simulink model "myMotor"  (R2020a)
settings: Solver=FixedStepAuto  StartTime=0.0  StopTime=10  FixedStep=0.005  RelTol=1e-3
values from neighbouring files (symbols this model uses):
  B = 6.60509857261e-05    [myNewMotor.mat]
  J = 3.18348551573e-05    [myNewMotor.mat]
  K = 0.0751678132976    [myNewMotor.mat]
  L = 0.0712541882931    [myNewMotor.mat]
  R = 6.4    [myNewMotor.mat]
settings Model: OrderedModelArguments=off  Creator=sabir  LastModifiedBy=sabir

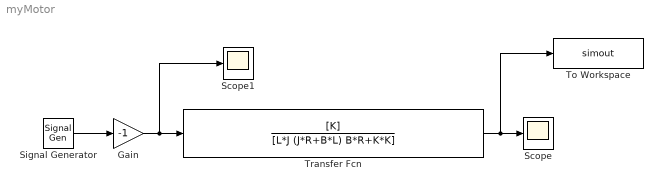
== system myMotor ==
  Gain : Gain  Gain=-1
  Scope : Scope
  Scope1 : Scope
  Signal Generator : SignalGenerator  WaveForm=square  Amplitude=24  Frequency=0.5
  To Workspace : ToWorkspace  VariableName=simout  SampleTime=-1
  Transfer Fcn : TransferFcn  Numerator=[K]  Denominator=[L*J (J*R+B*L) B*R+K*K]
  wires:
  Signal Generator/1 -> Gain/1
  Gain/1 -> Scope1/1, Transfer Fcn/1
  Transfer Fcn/1 -> To Workspace/1, Scope/1
